simulink model "KranAufg3"  (R2017a)
settings: Solver=ode5  StartTime=0  StopTime=10  FixedStep=T_S  RelTol=1e-3  EnableMultiTasking=on
undefined symbols (not defined in the file or in its folder): Crane3D_RangeBit, Crane3D_ScaleCoeff
undefined symbols (not defined in the file): rtdac4pciebaseaddress, T_S
settings Model: SimulationMode=external  ExtModeTrigDuration=30000  Creator=fbrombach  LastModifiedBy=hahn
settings DataIOCC: SaveFormat=Array
settings OptimizationCC: BooleanDataType=off  InitFltsAndDblsToZero=on
settings DebuggingCC: UnderspecifiedInitializationDetection=Classic  MergeDetectMultiDrivingBlocksExec=none  SolverPrmCheckMsg=warning  StateNameClashWarn=warning  SFUnexpectedBacktrackingDiag=warning  SFNoUnconditionalDefaultTransitionDiag=warning  SFExecutionAtInitializationDiag=none
settings ModelReferenceCC: PropagateSignalLabelsOutOfModel=off
settings RTWCC: SystemTargetFile=sldrt.tlc  TemplateMakefile=sldrt.tmf  Description=Simulink Desktop Real-Time  RTWCompilerOptimization=on
settings CodeAppCC: MaxIdLength=95
settings SimulinkDesktopRealTimeCC: TargetPreCompLibLocation=C:\Program Files\MATLAB\R2017a\toolbox\sldrt\lib\win64  TargetLangStandard=C89/C90 (ANSI)  SupportVariableSizeSignals=off
settings ConfigComp: CovMetricSettings=dw  CovHtmlReporting=on  CovSaveCumulativeToWorkspaceVar=on  CovSaveSingleToWorkspaceVar=on  CovExternalEMLEnable=off

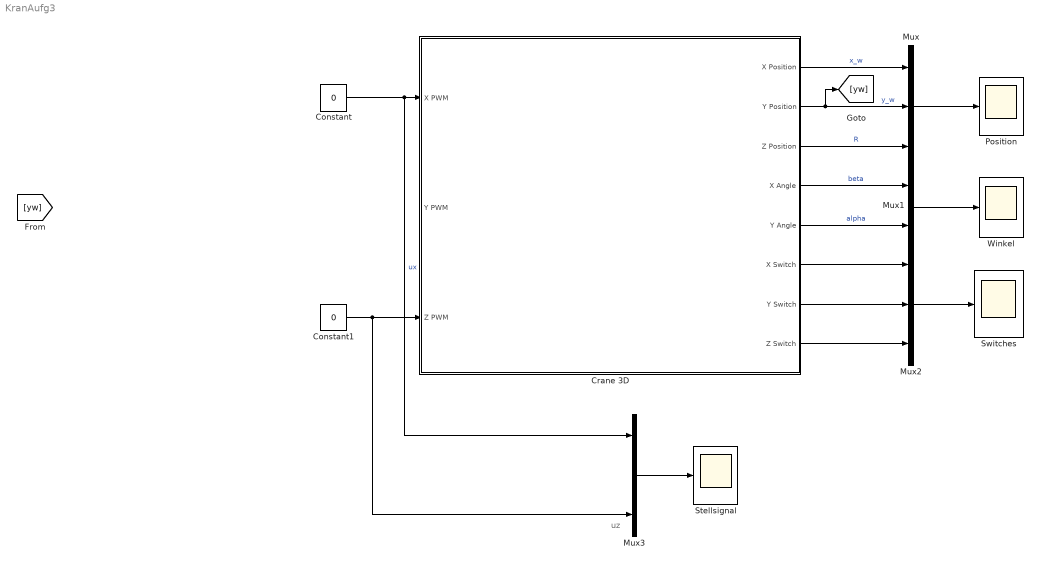
== system KranAufg3 ==
  note: uz
  Constant : Constant  Value=0
  Constant1 : Constant  Value=0
  Crane 3D : Subsystem  mask{BaseAddress=rtdac4pciebaseaddress, T0=T_S}
      mask prompts: BaseAddress "Base Address:"; T0 "Samping Period:"
      mask Display: image(imread('crane.jpeg'))
  Mux : Mux  Inputs=3
  Mux1 : Mux  Inputs=2
  Mux2 : Mux  Inputs=3
  Mux3 : Mux  Inputs=3
  Position : Scope
  Stellsignal : Scope
  Switches : Scope
  Winkel : Scope
  wires:
  Crane 3D/1(X Position) -> Mux/1  "x_w"
  Crane 3D/2(Y Position) -> Mux/2, [yw]  "y_w"
  Mux/1 -> Position/1
  Crane 3D/3(Z Position) -> Mux/3  "R"
  Crane 3D/4(X Angle) -> Mux1/1  "beta"
  Crane 3D/5(Y Angle) -> Mux1/2  "alpha"
  Mux1/1 -> Winkel/1
  Crane 3D/7(Y Switch) -> Mux2/2
  Crane 3D/8(Z Switch) -> Mux2/3
  Mux2/1 -> Switches/1
  Crane 3D/6(X Switch) -> Mux2/1
  Mux3/1 -> Stellsignal/1
  Constant1/1 -> Mux3/3, Crane 3D/3(Z PWM)
  ? -> Mux3/2, Crane 3D/2(Y PWM)  "uy"
  Constant/1 -> Mux3/1, Crane 3D/1(X PWM)  "ux"

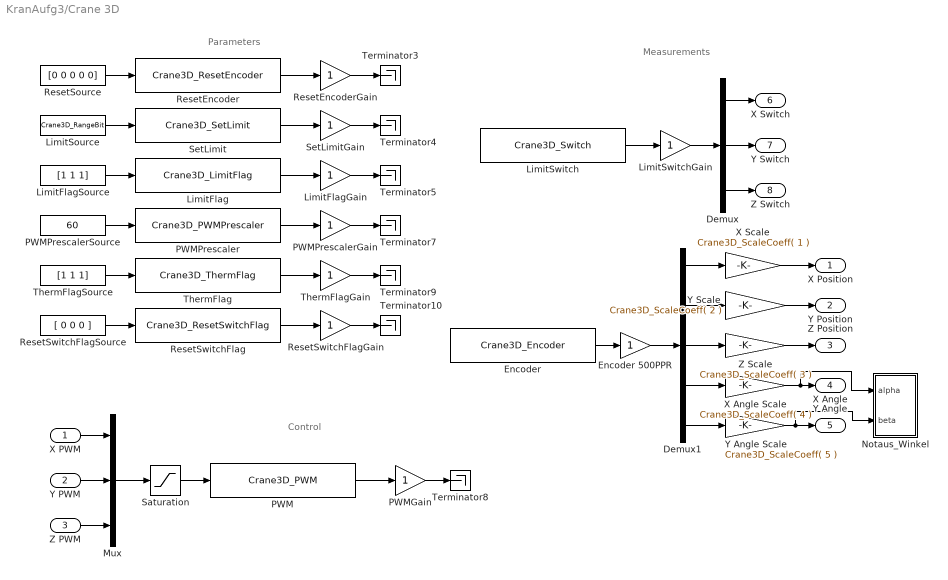
== system KranAufg3/Crane 3D ==
  note: Measurements
  note: Control
  note: Parameters
  X PWM : Inport
  Y PWM : Inport  Port=2
  Z PWM : Inport  Port=3
  Demux : Demux  Outputs=3
  Demux1 : Demux  Outputs=5
  Encoder : S-Function  FunctionName=Crane3D_Encoder  Parameters=BaseAddress, T0  SFunctionDeploymentMode=off  EnableBusSupport=off
  Encoder 500PPR : Gain  SaturateOnIntegerOverflow=on  OutDataTypeStr=Inherit: Same as input  ParamDataTypeStr=Inherit: Same as input
  LimitFlag : S-Function  FunctionName=Crane3D_LimitFlag  Parameters=BaseAddress, T0  SFunctionDeploymentMode=off  EnableBusSupport=off
  LimitFlagGain : Gain  SaturateOnIntegerOverflow=on  OutDataTypeStr=Inherit: Same as input  ParamDataTypeStr=Inherit: Same as input
  LimitFlagSource : Constant  Value=[1 1 1]
  LimitSource : Constant  Value=Crane3D_RangeBit
  LimitSwitch : S-Function  FunctionName=Crane3D_Switch  Parameters=BaseAddress, T0  SFunctionDeploymentMode=off  EnableBusSupport=off
  LimitSwitchGain : Gain  SaturateOnIntegerOverflow=on  OutDataTypeStr=Inherit: Same as input  ParamDataTypeStr=Inherit: Same as input
  Mux : Mux  Inputs=3
  Notaus_Winkel : Subsystem
  PWM : S-Function  FunctionName=Crane3D_PWM  Parameters=BaseAddress, T0  SFunctionDeploymentMode=off  EnableBusSupport=off
  PWMGain : Gain  SaturateOnIntegerOverflow=on  OutDataTypeStr=Inherit: Same as input  ParamDataTypeStr=Inherit: Same as input
  PWMPrescaler : S-Function  FunctionName=Crane3D_PWMPrescaler  Parameters=BaseAddress, T0  SFunctionDeploymentMode=off  EnableBusSupport=off
  PWMPrescalerGain : Gain  SaturateOnIntegerOverflow=on  OutDataTypeStr=Inherit: Same as input  ParamDataTypeStr=Inherit: Same as input
  PWMPrescalerSource : Constant  Value=60
  ResetEncoder : S-Function  FunctionName=Crane3D_ResetEncoder  Parameters=BaseAddress, T0  SFunctionDeploymentMode=off  EnableBusSupport=off
  ResetEncoderGain : Gain  SaturateOnIntegerOverflow=on  OutDataTypeStr=Inherit: Same as input  ParamDataTypeStr=Inherit: Same as input
  ResetSource : Constant  Value=[0 0 0 0 0]
  "ResetSwitchFlag " : S-Function  FunctionName=Crane3D_ResetSwitchFlag  Parameters=BaseAddress, T0  SFunctionDeploymentMode=off  EnableBusSupport=off
  ResetSwitchFlagGain : Gain  SaturateOnIntegerOverflow=on  OutDataTypeStr=Inherit: Same as input  ParamDataTypeStr=Inherit: Same as input
  ResetSwitchFlagSource : Constant  Value=[ 0 0 0 ]
  Saturation : Saturate  UpperLimit=1  LowerLimit=-1
  SetLimit : S-Function  FunctionName=Crane3D_SetLimit  Parameters=BaseAddress, T0  SFunctionDeploymentMode=off  EnableBusSupport=off
  SetLimitGain : Gain  SaturateOnIntegerOverflow=on  OutDataTypeStr=Inherit: Same as input  ParamDataTypeStr=Inherit: Same as input
  Terminator{3..5,7..10} (7 alike) : Terminator
  "ThermFlag " : S-Function  FunctionName=Crane3D_ThermFlag  Parameters=BaseAddress, T0  SFunctionDeploymentMode=off  EnableBusSupport=off
  ThermFlagGain : Gain  SaturateOnIntegerOverflow=on  OutDataTypeStr=Inherit: Same as input  ParamDataTypeStr=Inherit: Same as input
  ThermFlagSource : Constant  Value=[1 1 1]
  X Angle Scale : Gain  Gain=Crane3D_ScaleCoeff( 4 )  OutDataTypeStr=Inherit: Same as input  ParamDataTypeStr=Inherit: Same as input
  X Scale : Gain  Gain=Crane3D_ScaleCoeff( 1 )  OutDataTypeStr=Inherit: Same as input  ParamDataTypeStr=Inherit: Same as input
  Y Angle Scale : Gain  Gain=Crane3D_ScaleCoeff( 5 )  OutDataTypeStr=Inherit: Same as input  ParamDataTypeStr=Inherit: Same as input
  Y Scale : Gain  Gain=Crane3D_ScaleCoeff( 2 )  OutDataTypeStr=Inherit: Same as input  ParamDataTypeStr=Inherit: Same as input
  Z Scale : Gain  Gain=Crane3D_ScaleCoeff( 3 )  OutDataTypeStr=Inherit: Same as input  ParamDataTypeStr=Inherit: Same as input
  X Position : Outport  InitialOutput=0
  Y Position : Outport  Port=2  InitialOutput=0
  Z Position : Outport  Port=3  InitialOutput=0
  X Angle : Outport  Port=4  InitialOutput=0
  Y Angle : Outport  Port=5  InitialOutput=0
  X Switch : Outport  Port=6  InitialOutput=0
  Y Switch : Outport  Port=7  InitialOutput=0
  Z Switch : Outport  Port=8  InitialOutput=0
  wires:
  Demux1/1 -> X Scale/1
  Demux1/2 -> Y Scale/1
  Demux1/3 -> Z Scale/1
  Demux1/4 -> X Angle Scale/1
  Demux1/5 -> Y Angle Scale/1
  Y Angle Scale/1 -> Notaus_Winkel/2(beta), Y Angle/1
  Y Scale/1 -> Y Position/1
  X Scale/1 -> X Position/1
  Z Scale/1 -> Z Position/1
  Demux/3 -> Z Switch/1
  Demux/2 -> Y Switch/1
  Demux/1 -> X Switch/1
  LimitSwitchGain/1 -> Demux/1
  LimitSwitch/1 -> LimitSwitchGain/1
  X PWM/1 -> Mux/1
  Y PWM/1 -> Mux/2
  Z PWM/1 -> Mux/3
  ResetSwitchFlagGain/1 -> Terminator10/1
  ThermFlagGain/1 -> Terminator9/1
  PWMPrescalerGain/1 -> Terminator7/1
  LimitFlagGain/1 -> Terminator5/1
  SetLimitGain/1 -> Terminator4/1
  ResetEncoderGain/1 -> Terminator3/1
  ResetSwitchFlagSource/1 -> "ResetSwitchFlag "/1
  ThermFlagSource/1 -> "ThermFlag "/1
  PWMPrescalerSource/1 -> PWMPrescaler/1
  LimitFlagSource/1 -> LimitFlag/1
  LimitSource/1 -> SetLimit/1
  ResetSource/1 -> ResetEncoder/1
  "ResetSwitchFlag "/1 -> ResetSwitchFlagGain/1
  "ThermFlag "/1 -> ThermFlagGain/1
  PWMPrescaler/1 -> PWMPrescalerGain/1
  LimitFlag/1 -> LimitFlagGain/1
  SetLimit/1 -> SetLimitGain/1
  ResetEncoder/1 -> ResetEncoderGain/1
  PWMGain/1 -> Terminator8/1
  PWM/1 -> PWMGain/1
  Mux/1 -> Saturation/1
  Saturation/1 -> PWM/1
  Encoder/1 -> Encoder 500PPR/1
  Encoder 500PPR/1 -> Demux1/1
  X Angle Scale/1 -> Notaus_Winkel/1(alpha), X Angle/1

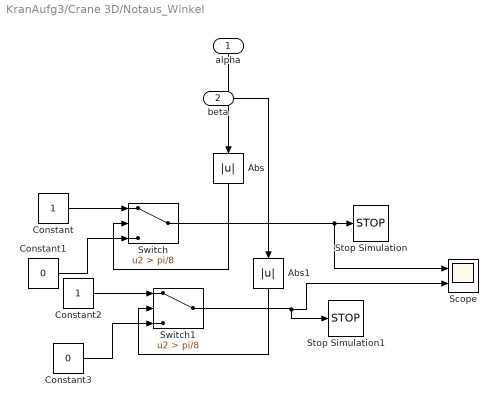
== system KranAufg3/Crane 3D/Notaus_Winkel ==
  alpha : Inport
  beta : Inport  Port=2
  Abs : Abs
  Abs1 : Abs
  Constant : Constant
  Constant1 : Constant  Value=0
  Constant2 : Constant
  Constant3 : Constant  Value=0
  Scope : Scope  NumInputPorts=2
  Stop Simulation : Stop
  Stop Simulation1 : Stop
  Switch : Switch  Criteria=u2 > Threshold  Threshold=pi/8
  Switch1 : Switch  Criteria=u2 > Threshold  Threshold=pi/8
  wires:
  alpha/1 -> Abs/1
  beta/1 -> Abs1/1
  Constant1/1 -> Switch/3
  Abs/1 -> Switch/2
  Switch1/1 -> Stop Simulation1/1, Scope/2
  Switch/1 -> Stop Simulation/1, Scope/1
  Constant2/1 -> Switch1/1
  Constant/1 -> Switch/1
  Constant3/1 -> Switch1/3
  Abs1/1 -> Switch1/2
